simulink model "OFDM_Transmitter_0621_3"  (R2020b)
settings: Solver=VariableStepAuto  StartTime=0.0  StopTime=10.0  RelTol=1e-3
undefined symbols (not defined in the file or in its folder): j
libraries: dspxfrm3 x1, commrandsrc3 x1, eeGeneralControl x1
settings Model: Creator=Lakshmi Mounika  LastModifiedBy=Lakshmi Mounika

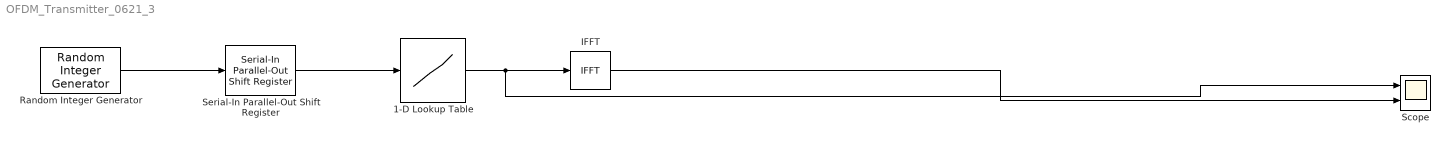
== system OFDM_Transmitter_0621_3 ==
  1-D Lookup Table : Lookup_n-D  NumberOfTableDimensions=1  BreakpointsForDimension1=[0 1 2 3]  Table=[1+j 1-j -1+j -1-j]  InternalRulePriority=Speed  RndMeth=Simplest  InputSameDT=on
  IFFT : dspxfrm3/IFFT  FFTImplementation=Auto  CompMethod=Table lookup  TableOpt=NEW  TableOptActive=Speed  BitRevOrder=off  cs_in=on  Normalize=on  InheritFFTLength=on  FFTLength=64  WrapInput=on  mode=Complex  outSamplingMode=Sample based  roundingMode=Floor  overflowMode=off  firstCoeffDataTypeStr=Inherit: Same word length as input  firstCoeffLastDataTypeStr=Inherit: Same word length as input  outputMin=[]  outputMax=[]
  Random Integer Generator : commrandsrc3/Random Integer Generator  SetSize=4  SeedSource=Auto  Seed=0  SampleTime=1  SamplesPerFrame=1  OutputDataType=double  SimulateUsing=Interpreted execution
  Scope : Scope  NumInputPorts=2
  Serial-In Parallel-Out Shift Register : eeGeneralControl/Serial-In Parallel-Out Shift Register  N=4  IC=0  Ts=-1
      settings: SourceProductBaseCode=PS
  wires:
  Serial-In Parallel-Out Shift Register/1 -> 1-D Lookup Table/1
  Random Integer Generator/1 -> Serial-In Parallel-Out Shift Register/1
  1-D Lookup Table/1 -> Scope/1, IFFT/1
  IFFT/1 -> Scope/2
